simulink model "clearing_faulted_segment_travelling_Wave"  (R2018a)
settings: Solver=ode23t  StartTime=0.0  StopTime=2  MaxStep=1e-3  RelTol=1e-3
values from neighbouring files (symbols this model uses):
  AC_lim = [1.5 -1.5]    [MT_HVDC_initialize.m]
  C_pm = 10.48e-3    (= 0.01048)    [MT_HVDC_initialize.m]
  ccsc_lim = [1.0 -1.0]    [MT_HVDC_initialize.m]
  DC_lim = [1.05 -1.05]    [MT_HVDC_initialize.m]
  f = 50    [MT_HVDC_initialize.m]
  Fc = 50    [MT_HVDC_initialize.m]
  Fn_filter = 1000    [MT_HVDC_initialize.m]
  Ireg_lim_i = [1.5, -1.5]    [MT_HVDC_initialize.m]
  Ireg_lim_r = [1.5, -1.5]    [MT_HVDC_initialize.m]
  Ki_ACreg_i = 260    [MT_HVDC_initialize.m]
  Ki_ccsc = 5    [MT_HVDC_initialize.m]
  Ki_DCreg_r = 150    [MT_HVDC_initialize.m]
  Ki_Ireg_i = 200    [MT_HVDC_initialize.m]
  Ki_Ireg_r = 100    [MT_HVDC_initialize.m]
  Ki_R_inv = 150000    [MT_HVDC_initialize.m]
  Ki_R_rec = 5000    [MT_HVDC_initialize.m]
  Kp_ACreg_i = 2    [MT_HVDC_initialize.m]
  Kp_ccsc = 1    [MT_HVDC_initialize.m]
  Kp_DCreg_r = 8    [MT_HVDC_initialize.m]
  Kp_Ireg_i = 2    [MT_HVDC_initialize.m]
  Kp_Ireg_r = 2    [MT_HVDC_initialize.m]
  Kp_R_inv = 0.001    [MT_HVDC_initialize.m]
  Kp_R_rec = 0.001    [MT_HVDC_initialize.m]
  L1_pu = 0.109    [MT_HVDC_initialize.m]
  L2_pu = 0.0824    [MT_HVDC_initialize.m]
  L_arm = L_arm_pu*Z_base66/w    [MT_HVDC_initialize.m]
  L_arm_pu = 0.15    [MT_HVDC_initialize.m]
  L_int = X_int/w    [MT_HVDC_initialize.m]
  n = 50    [MT_HVDC_initialize.m]
  n2 = 50    [MT_HVDC_initialize.m]
  P_nom = 220e6    (= 220000000)    [MT_HVDC_initialize.m]
  R1_pu = 0.00206    [MT_HVDC_initialize.m]
  R2_pu = 0.00206    [MT_HVDC_initialize.m]
  R_arm = 0.03    [MT_HVDC_initialize.m]
  R_arm_pu = R_arm/Z_base66    [MT_HVDC_initialize.m]
  R_int = sqrt((z_int_400^2)/(1+xr_ratio^2))    [MT_HVDC_initialize.m]
  Rg_T1 = 40    [MT_HVDC_initialize.m]
  S1_nom = P_nom    (= 220000000)    [MT_HVDC_initialize.m]
  S2_nom = P_nom    (= 220000000)    [MT_HVDC_initialize.m]
  T_fault = 1.4    [MT_HVDC_initialize.m]
  Ts_Control = 40e-6    (= 4e-05)    [MT_HVDC_initialize.m]
  Ts_Power = 20e-6    (= 2e-05)    [MT_HVDC_initialize.m]
  V1_prim = V_prim    (= 400000)    [MT_HVDC_initialize.m]
  V1_sec = V_grid    (= 66000)    [MT_HVDC_initialize.m]
  V2_prim = V_grid    (= 66000)    [MT_HVDC_initialize.m]
  V2_sec = 18e3    (= 18000)    [MT_HVDC_initialize.m]
  V_ac_ref = 1.035    [MT_HVDC_initialize.m]
  V_grid = 66e3    (= 66000)    [MT_HVDC_initialize.m]
  V_prim = 400e3    (= 400000)    [MT_HVDC_initialize.m]
  Vc_pm_r = 0*Vdc_nom/n    (= 0)    [MT_HVDC_initialize.m]
  Vdc_nom = 135e3    (= 135000)    [MT_HVDC_initialize.m]
  w = 2*pi*f    (= 314.159265359)    [MT_HVDC_initialize.m]
  z0z1 = 0.8    [MT_HVDC_initialize.m]
  Zeta_filter = 1    [MT_HVDC_initialize.m]
undefined symbols (not defined in the file or in its folder): D1, Delta, DiscIntNeverNeededParam
libraries: powerlib x417, powerlib_meascontrol x130, simulink x84, powerlib_extras x8, simulink_extras x5
(part 13 of 17)

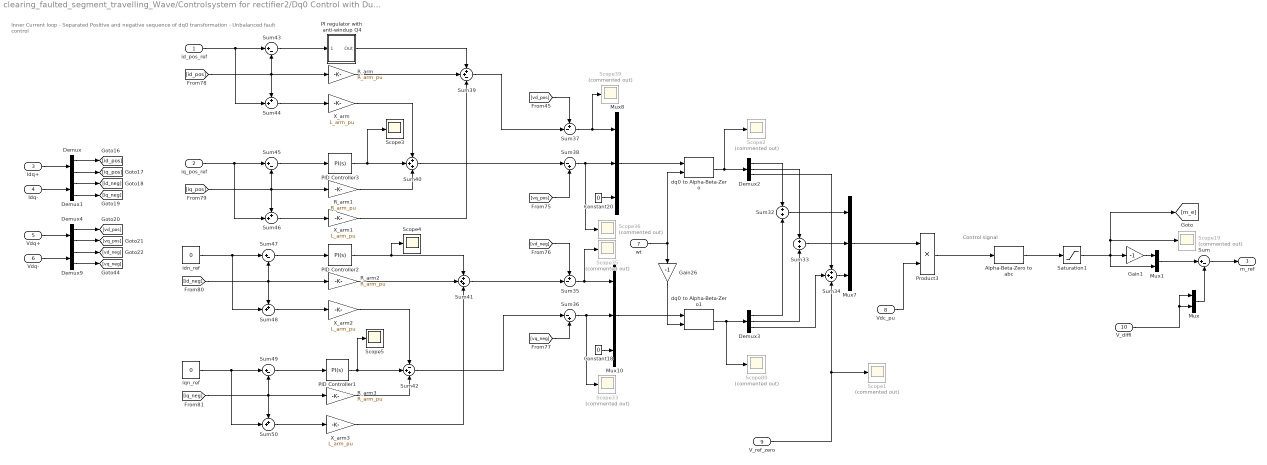
== system clearing_faulted_segment_travelling_Wave/Controlsystem for rectifier2/Dq0 Control with Dual Synchronous Reference Frame (DSRF)/Inner Current loop - Positive and Negative Sequence Control - Rectifier ==
  note: Control signal
  note: Inner Current loop - Separated Positive and negative sequence of dq0 transformation - Unbalanced fault control
  id_pos_ref : Inport
  iq_pos_ref : Inport  Port=2
  Idq+ : Inport  Port=3
  Idq- : Inport  Port=4
  Vdq+ : Inport  Port=5
  Vdq- : Inport  Port=6
  wt : Inport  Port=7
  Vdc_pu : Inport  Port=8
  V_ref_zero : Inport  Port=9
  V_diffi : Inport  Port=10
  Alpha-Beta-Zero to abc : powerlib_meascontrol/Transformations/Alpha-Beta-Zero to abc
      settings: SourceProductName=Simscape Electrical  SourceProductBaseCode=PS
  Constant18 : Constant  Value=0
  Constant20 : Constant  Value=0
  Demux{,1,4,9} (4 alike) : Demux  Outputs=2
  Demux2 : Demux  Outputs=3
  Demux3 : Demux  Outputs=3
  Gain1 : Gain  Gain=-1
  Gain26 : Gain  Gain=-1
  Mux : Mux  Inputs=2
  Mux1 : Mux  Inputs=2
  Mux10 : Mux  Inputs=3
  Mux7 : Mux  Inputs=3
  Mux8 : Mux  Inputs=3
  PI regulator with anti-windup Q4 : Subsystem  DialogController=POWERSYS.PowerSysDialog  mask(Discrete PI Controller){Kp=Kp_Ireg_r, Ki=Ki_Ireg_r, Par_Limits=[Ireg_lim_r(1) Ireg_lim_r(2)], Init=0, Ts=Ts_Control}
      mask prompts: Kp "Proportional gain (Kp):"; Ki "Integral gain (Ki):"; Par_Limits "Output limits: [ Upper   Lower ]"; Init "Output initial value:"; Ts "Sample time:"
      mask help: This block implements a discrete PI controller.
      mask init:
      | UpperLimit=Par_Limits(1);
      | LowerLimit=Par_Limits(2);
      | power_initmask();
      mask Help: This block is part of a subset of blocks in the Extras library that does not have documentation associated with it, other than the block mask description.
      mask Display: disp('PI');
  PID Controller1 : simulink/Continuous/PID Controller  Controller=PI  TimeDomain=Continuous-time  SampleTime=-1  IntegratorMethod=Forward Euler  FilterMethod=Forward Euler  Form=Parallel  UseFilter=on  ControllerParametersSource=internal  P=Kp_Ireg_r*0.5  I=Ki_Ireg_r*0.5  D=0  N=100  InitialConditionSource=internal  InitialConditionForIntegrator=0  InitialConditionForFilter=0  ExternalReset=none  LimitOutput=off  UpperSaturationLimit=inf  LowerSaturationLimit=-inf  LinearizeAsGain=on  AntiWindupMode=none  Kb=1  TrackingMode=off  Kt=1  PParamMin=[]  PParamMax=[]  IParamMin=[]  IParamMax=[]  DParamMin=[]  DParamMax=[]  NParamMin=[]  NParamMax=[]  KbParamMin=[]  KbParamMax=[]  KtParamMin=[]  KtParamMax=[]  POutMin=[]  POutMax=[]  IOutMin=[]  IOutMax=[]  DOutMin=[]  DOutMax=[]  NOutMin=[]  NOutMax=[]  KbOutMin=[]  KbOutMax=[]  KtOutMin=[]  KtOutMax=[]  IntegratorOutMin=[]  IntegratorOutMax=[]  FilterOutMin=[]  FilterOutMax=[]  SumOutMin=[]  SumOutMax=[]  SumI1OutMin=[]  SumI1OutMax=[]  SumI2OutMin=[]  SumI2OutMax=[]  SumI3OutMin=[]  SumI3OutMax=[]  SumDOutMin=[]  SumDOutMax=[]  SaturationOutMin=[]  SaturationOutMax=[]  IntegratorContinuousStateAttributes=''  IntegratorStateMustResolveToSignalObject=off  IntegratorRTWStateStorageClass=Auto  FilterContinuousStateAttributes=''  FilterStateMustResolveToSignalObject=off  FilterRTWStateStorageClass=Auto  DifferentiatorICPrevScaledInput=0  DifferentiatorOutMin=[]  DifferentiatorOutMax=[]  FilterDiffOutCoefMin=[]  FilterDiffOutCoefMax=[]  SumDenOutMin=[]  SumDenOutMax=[]  SumNumOutMin=[]  SumNumOutMax=[]  ReciprocalOutMin=[]  ReciprocalOutMax=[]  DivideOutMin=[]  DivideOutMax=[]  TunerSelectOption=Transfer Function Based (PID Tuner App)
  PID Controller2 : simulink/Continuous/PID Controller  Controller=PI  TimeDomain=Continuous-time  SampleTime=-1  IntegratorMethod=Forward Euler  FilterMethod=Forward Euler  Form=Parallel  UseFilter=on  ControllerParametersSource=internal  P=Kp_Ireg_r*0.5  I=Ki_Ireg_r*0.5  D=0  N=100  InitialConditionSource=internal  InitialConditionForIntegrator=0  InitialConditionForFilter=0  ExternalReset=none  LimitOutput=off  UpperSaturationLimit=inf  LowerSaturationLimit=-inf  LinearizeAsGain=on  AntiWindupMode=none  Kb=1  TrackingMode=off  Kt=1  PParamMin=[]  PParamMax=[]  IParamMin=[]  IParamMax=[]  DParamMin=[]  DParamMax=[]  NParamMin=[]  NParamMax=[]  KbParamMin=[]  KbParamMax=[]  KtParamMin=[]  KtParamMax=[]  POutMin=[]  POutMax=[]  IOutMin=[]  IOutMax=[]  DOutMin=[]  DOutMax=[]  NOutMin=[]  NOutMax=[]  KbOutMin=[]  KbOutMax=[]  KtOutMin=[]  KtOutMax=[]  IntegratorOutMin=[]  IntegratorOutMax=[]  FilterOutMin=[]  FilterOutMax=[]  SumOutMin=[]  SumOutMax=[]  SumI1OutMin=[]  SumI1OutMax=[]  SumI2OutMin=[]  SumI2OutMax=[]  SumI3OutMin=[]  SumI3OutMax=[]  SumDOutMin=[]  SumDOutMax=[]  SaturationOutMin=[]  SaturationOutMax=[]  IntegratorContinuousStateAttributes=''  IntegratorStateMustResolveToSignalObject=off  IntegratorRTWStateStorageClass=Auto  FilterContinuousStateAttributes=''  FilterStateMustResolveToSignalObject=off  FilterRTWStateStorageClass=Auto  DifferentiatorICPrevScaledInput=0  DifferentiatorOutMin=[]  DifferentiatorOutMax=[]  FilterDiffOutCoefMin=[]  FilterDiffOutCoefMax=[]  SumDenOutMin=[]  SumDenOutMax=[]  SumNumOutMin=[]  SumNumOutMax=[]  ReciprocalOutMin=[]  ReciprocalOutMax=[]  DivideOutMin=[]  DivideOutMax=[]  TunerSelectOption=Transfer Function Based (PID Tuner App)
  PID Controller3 : simulink/Continuous/PID Controller  Controller=PI  TimeDomain=Continuous-time  SampleTime=-1  IntegratorMethod=Forward Euler  FilterMethod=Forward Euler  Form=Parallel  UseFilter=on  ControllerParametersSource=internal  P=Kp_Ireg_r  I=Ki_Ireg_r  D=0  N=100  InitialConditionSource=internal  InitialConditionForIntegrator=0  InitialConditionForFilter=0  ExternalReset=none  LimitOutput=off  UpperSaturationLimit=inf  LowerSaturationLimit=-inf  LinearizeAsGain=on  AntiWindupMode=none  Kb=1  TrackingMode=off  Kt=1  PParamMin=[]  PParamMax=[]  IParamMin=[]  IParamMax=[]  DParamMin=[]  DParamMax=[]  NParamMin=[]  NParamMax=[]  KbParamMin=[]  KbParamMax=[]  KtParamMin=[]  KtParamMax=[]  POutMin=[]  POutMax=[]  IOutMin=[]  IOutMax=[]  DOutMin=[]  DOutMax=[]  NOutMin=[]  NOutMax=[]  KbOutMin=[]  KbOutMax=[]  KtOutMin=[]  KtOutMax=[]  IntegratorOutMin=[]  IntegratorOutMax=[]  FilterOutMin=[]  FilterOutMax=[]  SumOutMin=[]  SumOutMax=[]  SumI1OutMin=[]  SumI1OutMax=[]  SumI2OutMin=[]  SumI2OutMax=[]  SumI3OutMin=[]  SumI3OutMax=[]  SumDOutMin=[]  SumDOutMax=[]  SaturationOutMin=[]  SaturationOutMax=[]  IntegratorContinuousStateAttributes=''  IntegratorStateMustResolveToSignalObject=off  IntegratorRTWStateStorageClass=Auto  FilterContinuousStateAttributes=''  FilterStateMustResolveToSignalObject=off  FilterRTWStateStorageClass=Auto  DifferentiatorICPrevScaledInput=0  DifferentiatorOutMin=[]  DifferentiatorOutMax=[]  FilterDiffOutCoefMin=[]  FilterDiffOutCoefMax=[]  SumDenOutMin=[]  SumDenOutMax=[]  SumNumOutMin=[]  SumNumOutMax=[]  ReciprocalOutMin=[]  ReciprocalOutMax=[]  DivideOutMin=[]  DivideOutMax=[]  TunerSelectOption=Transfer Function Based (PID Tuner App)
  Product3 : Product
  R_arm{,1..3} (4 alike) : Gain  Gain=R_arm_pu
  Saturation1 : Saturate  UpperLimit=Ireg_lim_r(1) + 1.1*0  LowerLimit=Ireg_lim_r(2)
  Scope{1..2,19,33,35..36,39,80} (8 alike) : Scope  Commented=on
  Scope3 : Scope
  Scope4 : Scope
  Scope5 : Scope
  Sum{,43,45,47,49} (5 alike) : Sum  Inputs=|+-
  Sum32 : Sum
  Sum33 : Sum
  Sum34 : Sum  Inputs=+++
  Sum35 : Sum  Inputs=+-|
  Sum36 : Sum  Inputs=|-+
  Sum37 : Sum  Inputs=+-|
  Sum38 : Sum  Inputs=|-+
  Sum39 : Sum  Inputs=++-
  Sum40 : Sum  Inputs=+++
  Sum41 : Sum  Inputs=+++
  Sum42 : Sum  Inputs=-++
  Sum{44,46,48,50} (4 alike) : Sum  Inputs=++|
  X_arm{,1..3} (4 alike) : Gain  Gain=L_arm_pu
  dq0 to Alpha-Beta-Zero : powerlib_meascontrol/Transformations/dq0 to Alpha-Beta-Zero  Alignment=90 degrees behind phase A axis
      settings: SourceProductName=Simscape Electrical  SourceProductBaseCode=PS
  dq0 to Alpha-Beta-Zero1 : powerlib_meascontrol/Transformations/dq0 to Alpha-Beta-Zero  Alignment=90 degrees behind phase A axis
      settings: SourceProductName=Simscape Electrical  SourceProductBaseCode=PS
  idn_ref : Constant  Value=0
  iqn_ref : Constant  Value=0
  m_ref : Outport
  wires:
  Vdq-/1 -> Demux9/1
  Idq-/1 -> Demux1/1
  Vdq+/1 -> Demux4/1
  Demux9/2 -> [vq_neg]
  Demux1/1 -> [id_neg]
  Demux4/2 -> [vq_pos]
  Demux4/1 -> [vd_pos]
  Demux/1 -> [id_pos]
  Demux/2 -> [iq_pos]
  wt/1 -> Gain26/1, dq0 to Alpha-Beta-Zero/2
  Sum36/1 -> Mux10/2, Scope33/1
  Sum45/1 -> PID Controller3/1
  Sum37/1 -> Mux8/1, Scope39/1
  V_ref_zero/1 -> Scope1/1, Sum34/3
  X_arm3/1 -> Sum41/3
  X_arm2/1 -> Sum42/1
  iq_pos_ref/1 -> Sum45/1, Sum46/2
  idn_ref/1 -> Sum47/1, Sum48/2
  Demux3/1 -> Sum32/2
  Sum40/1 -> Sum38/1
  X_arm1/1 -> Sum39/3
  [vq_neg] -> Sum36/2
  R_arm1/1 -> Sum40/3
  Sum48/1 -> X_arm2/1
  R_arm/1 -> Sum39/2
  Sum44/1 -> X_arm/1
  Sum43/1 -> PI regulator with anti-windup Q4/1(Error)
  Sum46/1 -> X_arm1/1
  Product3/1 -> Alpha-Beta-Zero to abc/1
  Sum38/1 -> Scope36/1, Mux8/2
  [vd_pos] -> Sum37/1
  iqn_ref/1 -> Sum49/1, Sum50/2
  Idq+/1 -> Demux/1
  [vd_neg] -> Sum35/1
  Sum47/1 -> PID Controller2/1
  [vq_pos] -> Sum38/2
  X_arm/1 -> Sum40/1
  Sum33/1 -> Mux7/2
  R_arm3/1 -> Sum42/3
  Sum41/1 -> Sum35/2
  Demux2/1 -> Sum32/1
  Sum42/1 -> Sum36/1
  Sum39/1 -> Sum37/2
  id_pos_ref/1 -> Sum43/1, Sum44/2
  [iq_neg] -> Sum49/2, Sum50/1, R_arm3/1
  Demux3/3 -> Sum34/2
  [id_neg] -> Sum48/1, Sum47/2, R_arm2/1
  Sum35/1 -> Mux10/1, Scope35/1
  [id_pos] -> Sum44/1, Sum43/2, R_arm/1
  Constant20/1 -> Mux8/3
  Constant18/1 -> Mux10/3
  Demux2/2 -> Sum33/1
  Demux2/3 -> Sum34/1
  Sum50/1 -> X_arm3/1
  Sum49/1 -> PID Controller1/1
  [iq_pos] -> Sum45/2, Sum46/1, R_arm1/1
  Sum34/1 -> Mux7/3
  Demux3/2 -> Sum33/2
  R_arm2/1 -> Sum41/2
  dq0 to Alpha-Beta-Zero/1 -> Demux2/1, Scope2/1
  Sum32/1 -> Mux7/1
  Gain26/1 -> dq0 to Alpha-Beta-Zero1/2
  Demux1/2 -> [iq_neg]
  dq0 to Alpha-Beta-Zero1/1 -> Demux3/1, Scope80/1
  Demux9/1 -> [vd_neg]
  Alpha-Beta-Zero to abc/1 -> Saturation1/1
  Mux10/1 -> dq0 to Alpha-Beta-Zero1/1
  Mux8/1 -> dq0 to Alpha-Beta-Zero/1
  Mux7/1 -> Product3/1
  Vdc_pu/1 -> Product3/2
  PID Controller3/1 -> Sum40/2, Scope3/1
  PID Controller2/1 -> Sum41/1, Scope4/1
  PID Controller1/1 -> Sum42/2, Scope5/1
  PI regulator with anti-windup Q4/1(Out) -> Sum39/1
  V_diffi/1 -> Mux/1, Mux/2
  Mux/1 -> Sum/2
  Mux1/1 -> Sum/1
  Sum/1 -> m_ref/1
  Saturation1/1 -> Gain1/1, Mux1/2, Scope19/1, [m_e]
  Gain1/1 -> Mux1/1

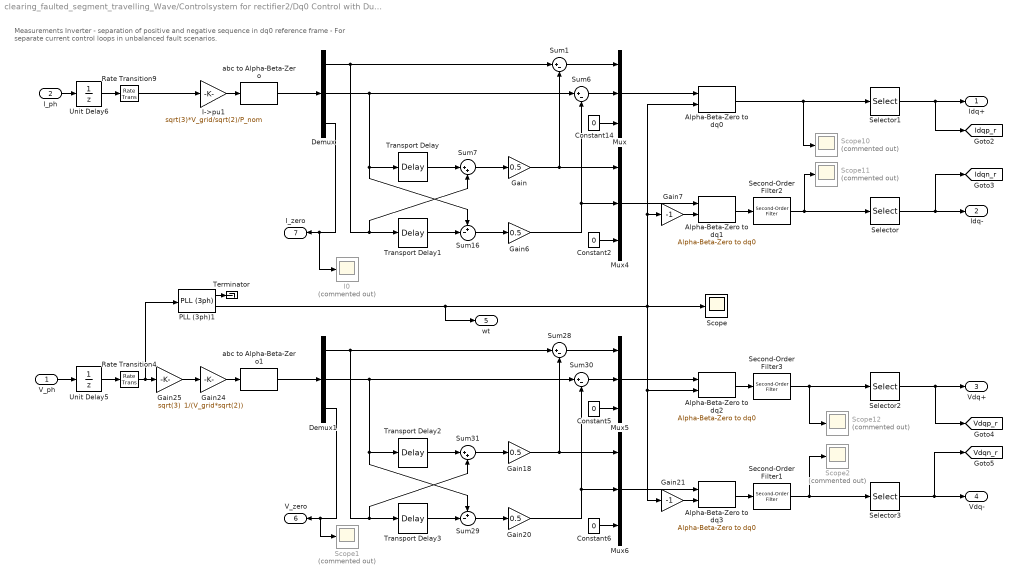
== system clearing_faulted_segment_travelling_Wave/Controlsystem for rectifier2/Dq0 Control with Dual Synchronous Reference Frame (DSRF)/Measurement - dq0 positiveand negative sequence, - and zero sequence in alphabetta - Rectifier ==
  note: Measurements Inverter - separation of positive and negative sequence in dq0 reference frame - For separate current control loops in unbalanced fault scenarios.
  V_ph : Inport
  I_ph : Inport  Port=2
  Alpha-Beta-Zero to dq{0..3} (4 alike) : powerlib_meascontrol/Transformations/Alpha-Beta-Zero to dq0  Alignment=90 degrees behind phase A axis
      settings: SourceProductName=Simscape Electrical
  Constant{2,5..6,14} (4 alike) : Constant  Value=0
  Demux : Demux  Outputs=3
  Demux1 : Demux  Outputs=3
  Gain{,6,18,20} (4 alike) : Gain  Gain=0.5
  Gain21 : Gain  Gain=-1
  Gain24 : Gain  Gain=1/(V_grid*sqrt(2))
  Gain25 : Gain  Gain=sqrt(3)
  Gain7 : Gain  Gain=-1
  I->pu1 : Gain  Gain=sqrt(3)*V_grid/sqrt(2)/P_nom  SaturateOnIntegerOverflow=on  OutDataTypeStr=Inherit: Same as input  ParamDataTypeStr=Inherit: Same as input
  "I0 " : Scope  Commented=on
  Mux{,4..6} (4 alike) : Mux  Inputs=3
  PLL (3ph)1 : powerlib_meascontrol/PLL/PLL (3ph)  Fmin=45  Par_Init=[V_grid, f]  ParK=[180, 3200, 1]  TcD=1e-4  MaxRateChangeFreq=12  FilterCutOffFreq=25  Ts=0  AGC=on
      settings: SourceProductName=Simscape Electrical
  Rate Transition4 : RateTransition  OutPortSampleTime=Ts_Control
  Rate Transition9 : RateTransition  OutPortSampleTime=Ts_Control
  Scope : Scope
  Scope{1..2,10..12} (5 alike) : Scope  Commented=on
  Second-Order Filter1 : powerlib_meascontrol/Filters/Second-Order Filter  FilterType=Bandstop (Notch)  Fo=100  Zeta=Zeta_filter*0.8  Ts=Ts_Control  Initialize=off  Vac_Init="[0,  0,  60]"  Vdc_Init=0  PlotResponse=off  FreqRange=[0, 500, 1]
      settings: SourceProductName=Simscape Electrical  SourceProductBaseCode=PS
  Second-Order Filter2 : powerlib_meascontrol/Filters/Second-Order Filter  FilterType=Bandstop (Notch)  Fo=100  Zeta=Zeta_filter*0.8  Ts=Ts_Control  Initialize=off  Vac_Init="[0,  0,  60]"  Vdc_Init=0  PlotResponse=off  FreqRange=[0, 500, 1]
      settings: SourceProductName=Simscape Electrical  SourceProductBaseCode=PS
  Second-Order Filter3 : powerlib_meascontrol/Filters/Second-Order Filter  FilterType=Lowpass  Fo=Fn_filter  Zeta=Zeta_filter  Ts=Ts_Control  Initialize=off  Vac_Init="[0,  0,  60]"  Vdc_Init=0  PlotResponse=off  FreqRange=[0, 500, 1]
      settings: SourceProductName=Simscape Electrical  SourceProductBaseCode=PS
  Selector{,1..3} (4 alike) : Selector  InputPortWidth=3  IndexOptions=Index vector (dialog)  Indices=[1 2]  OutputSizes=1
  Sum{1,6,28,30} (4 alike) : Sum  Inputs=|+-
  Sum16 : Sum  Inputs=+-|
  Sum29 : Sum  Inputs=+-|
  Sum31 : Sum  Inputs=|++
  Sum7 : Sum  Inputs=|++
  Terminator : Terminator
  Transport Delay{,1..3} (4 alike) : TransportDelay  DelayTime=1/(f*4)  BufferSize=1024*15
  Unit Delay5 : UnitDelay  SampleTime=Ts_Power
  Unit Delay6 : UnitDelay  SampleTime=Ts_Power
  abc to Alpha-Beta-Zero : powerlib_meascontrol/Transformations/abc to Alpha-Beta-Zero
      settings: SourceProductName=Simscape Electrical
  abc to Alpha-Beta-Zero1 : powerlib_meascontrol/Transformations/abc to Alpha-Beta-Zero
      settings: SourceProductName=Simscape Electrical
  Idq+ : Outport
  Idq- : Outport  Port=2
  Vdq+ : Outport  Port=3
  Vdq- : Outport  Port=4
  wt : Outport  Port=5
  V_zero : Outport  Port=6
  I_zero : Outport  Port=7
  tag scope: Idqn_r=global, Idqp_r=global, Vdqn_r=global, Vdqp_r=global
  wires:
  Selector2/1 -> [Vdqp_r], Vdq+/1
  Selector1/1 -> [Idqp_r], Idq+/1
  Sum29/1 -> Gain20/1
  Constant6/1 -> Mux6/3
  Sum1/1 -> Mux/1
  Sum7/1 -> Gain/1
  Gain7/1 -> Alpha-Beta-Zero to dq1/2
  Gain21/1 -> Alpha-Beta-Zero to dq3/2
  I_ph/1 -> Unit Delay6/1
  Sum30/1 -> Mux5/2
  Demux/3 -> "I0 "/1, I_zero/1
  Mux4/1 -> Alpha-Beta-Zero to dq1/1
  Rate Transition9/1 -> I->pu1/1
  Transport Delay3/1 -> Sum29/2
  Demux/2 -> Sum6/1, Transport Delay/1, Sum16/1
  Constant2/1 -> Mux4/3
  Gain25/1 -> Gain24/1
  Gain24/1 -> abc to Alpha-Beta-Zero1/1
  I->pu1/1 -> abc to Alpha-Beta-Zero/1
  Unit Delay6/1 -> Rate Transition9/1
  Sum31/1 -> Gain18/1
  Unit Delay5/1 -> Rate Transition4/1
  Mux5/1 -> Alpha-Beta-Zero to dq2/1
  Sum28/1 -> Mux5/1
  Transport Delay2/1 -> Sum31/1
  Gain20/1 -> Sum30/2, Mux6/2
  Constant5/1 -> Mux5/3
  Mux6/1 -> Alpha-Beta-Zero to dq3/1
  Transport Delay/1 -> Sum7/1
  Sum6/1 -> Mux/2
  Gain18/1 -> Sum28/2, Mux6/1
  Gain/1 -> Mux4/1, Sum1/2
  Gain6/1 -> Mux4/2, Sum6/2
  Demux/1 -> Sum1/1, Sum7/2, Transport Delay1/1
  Demux1/3 -> Scope1/1, V_zero/1
  Transport Delay1/1 -> Sum16/2
  Mux/1 -> Alpha-Beta-Zero to dq0/1
  abc to Alpha-Beta-Zero/1 -> Demux/1
  Demux1/1 -> Transport Delay3/1, Sum31/2, Sum28/1
  abc to Alpha-Beta-Zero1/1 -> Demux1/1
  Demux1/2 -> Sum29/1, Transport Delay2/1, Sum30/1
  Sum16/1 -> Gain6/1
  Constant14/1 -> Mux/3
  Rate Transition4/1 -> PLL (3ph)1/1, Gain25/1
  PLL (3ph)1/2 -> wt/1, Gain7/1, Alpha-Beta-Zero to dq0/2, Scope/1, Alpha-Beta-Zero to dq2/2, Gain21/1
  V_ph/1 -> Unit Delay5/1
  PLL (3ph)1/1 -> Terminator/1
  Alpha-Beta-Zero to dq3/1 -> Second-Order Filter1/1
  Alpha-Beta-Zero to dq1/1 -> Second-Order Filter2/1
  Selector3/1 -> [Vdqn_r], Vdq-/1
  Selector/1 -> [Idqn_r], Idq-/1
  Alpha-Beta-Zero to dq0/1 -> Scope10/1, Selector1/1
  Alpha-Beta-Zero to dq2/1 -> Second-Order Filter3/1
  Second-Order Filter1/1 -> Scope2/1, Selector3/1
  Second-Order Filter3/1 -> Selector2/1, Scope12/1
  Second-Order Filter2/1 -> Scope11/1, Selector/1

== system clearing_faulted_segment_travelling_Wave/Controlsystem for rectifier2/Dq0 Control with Dual Synchronous Reference Frame (DSRF)/PWM Signal Generator - Rectifier ==
  U_ref : Inport
  Block : Inport  Port=2
  Add{,7..11} (6 alike) : Sum  Inputs=1
  Constant{3..8} (6 alike) : Constant  Value=0
  Constant9 : Constant  Value=[ 0, n ]
  Demux : Demux  Outputs=2
  Demux1 : Demux  Outputs=3
  Demux4 : Demux  Outputs=3
  Mux{7..12} (6 alike) : Mux  Inputs=2
  Mux13 : Mux  Inputs=6
  PWM Gen1 : Subsystem  mask(PWM generator for half-bridge MMC){n=n, Fc=Fc, Ts=Ts_Power}
      mask prompts: n "Number of half-bridges"; Fc "Carriers frequency (Hz)"; Ts "Sample time (s)"
      mask init: same as clearing_faulted_segment_travelling_Wave/Controlsystem for Inverter/Dq0 Control/PWM Signal Generator - Inverter1/PWM Gen1
  PWM Gen2 : Subsystem  mask(PWM generator for half-bridge MMC){n=n, Fc=Fc, Ts=Ts_Power}
      mask prompts: n "Number of half-bridges"; Fc "Carriers frequency (Hz)"; Ts "Sample time (s)"
      mask init: same as clearing_faulted_segment_travelling_Wave/Controlsystem for Inverter/Dq0 Control/PWM Signal Generator - Inverter1/PWM Gen1
  PWM Gen3 : Subsystem  mask(PWM generator for half-bridge MMC){n=n, Fc=Fc, Ts=Ts_Power}
      mask prompts: n "Number of half-bridges"; Fc "Carriers frequency (Hz)"; Ts "Sample time (s)"
      mask init: same as clearing_faulted_segment_travelling_Wave/Controlsystem for Inverter/Dq0 Control/PWM Signal Generator - Inverter1/PWM Gen1
  PWM Gen4 : Subsystem  mask(PWM generator for half-bridge MMC){n=n, Fc=Fc, Ts=Ts_Power}
      mask prompts: n "Number of half-bridges"; Fc "Carriers frequency (Hz)"; Ts "Sample time (s)"
      mask init: same as clearing_faulted_segment_travelling_Wave/Controlsystem for Inverter/Dq0 Control/PWM Signal Generator - Inverter1/PWM Gen1
  PWM Gen5 : Subsystem  mask(PWM generator for half-bridge MMC){n=n, Fc=Fc, Ts=Ts_Power}
      mask prompts: n "Number of half-bridges"; Fc "Carriers frequency (Hz)"; Ts "Sample time (s)"
      mask init: same as clearing_faulted_segment_travelling_Wave/Controlsystem for Inverter/Dq0 Control/PWM Signal Generator - Inverter1/PWM Gen1
  PWM Gen6 : Subsystem  mask(PWM generator for half-bridge MMC){n=n, Fc=Fc, Ts=Ts_Power}
      mask prompts: n "Number of half-bridges"; Fc "Carriers frequency (Hz)"; Ts "Sample time (s)"
      mask init: same as clearing_faulted_segment_travelling_Wave/Controlsystem for Inverter/Dq0 Control/PWM Signal Generator - Inverter1/PWM Gen1
  Selector{,1..5} (6 alike) : Selector  InputPortWidth=n*2  IndexOptions=Index vector (dialog)  Indices=[1:2:(n*2-1)]  OutputSizes=1
  Switch{,1..5} (6 alike) : Switch  Criteria=u2 ~= 0
  Terminator{,1..5} (6 alike) : Terminator
  g : Outport
  wires:
  Selector5/1 -> Add11/1
  Switch3/1 -> Mux13/4
  Switch4/1 -> Mux13/5
  PWM Gen1/1(P) -> Selector/1
  Demux4/3 -> PWM Gen3/1(Uref)
  Switch2/1 -> Mux13/3
  PWM Gen4/2(Cr) -> Terminator4/1
  Switch/1 -> Mux13/1
  Mux13/1 -> g/1
  Constant4/1 -> Mux8/2
  Demux1/3 -> PWM Gen6/1(Uref)
  Mux10/1 -> Switch3/3
  Mux8/1 -> Switch1/3
  Selector3/1 -> Add9/1
  Constant8/1 -> Mux12/2
  Selector4/1 -> Add10/1
  Constant6/1 -> Mux10/2
  Constant5/1 -> Mux9/2
  Selector1/1 -> Add7/1
  Demux1/1 -> PWM Gen4/1(Uref)
  Add9/1 -> Mux10/1
  Demux4/1 -> PWM Gen1/1(Uref)
  Selector2/1 -> Add8/1
  Add7/1 -> Mux8/1
  Constant9/1 -> Switch/1, Switch5/1, Switch4/1, Switch3/1, Switch2/1, Switch1/1
  PWM Gen3/2(Cr) -> Terminator1/1
  PWM Gen5/1(P) -> Selector4/1
  Constant7/1 -> Mux11/2
  Demux4/2 -> PWM Gen2/1(Uref)
  Mux12/1 -> Switch5/3
  PWM Gen6/2(Cr) -> Terminator3/1
  PWM Gen2/2(Cr) -> Terminator/1
  Switch5/1 -> Mux13/6
  Selector/1 -> Add/1
  Block/1 -> Switch/2, Switch1/2, Switch2/2, Switch3/2, Switch4/2, Switch5/2
  Add10/1 -> Mux11/1
  PWM Gen5/2(Cr) -> Terminator2/1
  Add11/1 -> Mux12/1
  Demux1/2 -> PWM Gen5/1(Uref)
  Mux11/1 -> Switch4/3
  Mux7/1 -> Switch/3
  Switch1/1 -> Mux13/2
  Constant3/1 -> Mux7/2
  PWM Gen4/1(P) -> Selector3/1
  PWM Gen2/1(P) -> Selector1/1
  Mux9/1 -> Switch2/3
  PWM Gen3/1(P) -> Selector2/1
  Add8/1 -> Mux9/1
  Add/1 -> Mux7/1
  PWM Gen6/1(P) -> Selector5/1
  PWM Gen1/2(Cr) -> Terminator5/1
  U_ref/1 -> Demux/1
  Demux/1 -> Demux4/1
  Demux/2 -> Demux1/1

== system clearing_faulted_segment_travelling_Wave/Controlsystem for rectifier2/Dq0 Control with Dual Synchronous Reference Frame (DSRF)/Zero Sequence Controller2 ==
  note: PR Controller
  V0_meas : Inport
  I0_meas : Inport  Port=2
  Enable : Inport  Port=3
  Enable1 : EnablePort
  Constant : Constant  Value=0
  Constant1 : Constant  Value=0
  I0_r_ref : Constant  Value=0
  Ki_R : Gain  Gain=Ki_R_rec
  Kp_R : Gain  Gain=Kp_R_rec
  Second-Order Filter1 : powerlib_meascontrol/Filters/Second-Order Filter  FilterType=Lowpass  Fo=f*4  Zeta=0.707  Ts=0  Initialize=on  Vac_Init="[0,  0,  60]"  Vdc_Init=0  PlotResponse=off  FreqRange=[0, 500, 1]
      settings: SourceProductName=Simscape Electrical  SourceProductBaseCode=PS
  Second-Order Filter2 : powerlib_meascontrol/Filters/Second-Order Filter  FilterType=Bandstop (Notch)  Fo=f*2  Zeta=0.707  Ts=0  Initialize=off  Vac_Init="[0,  0,  60]"  Vdc_Init=0  PlotResponse=off  FreqRange=[0, 500, 1]
      settings: SourceProductName=Simscape Electrical  SourceProductBaseCode=PS
  Sum2 : Sum  Inputs=+-|
  Sum3 : Sum  Inputs=++|
  Sum96 : Sum  Inputs=|++
  Switch : Switch  Criteria=u2 > Threshold
  Switch1 : Switch  Criteria=u2 > Threshold
  Transfer Fcn1 : TransferFcn  Denominator=[1 0 98596]
  V_zero_ref : Outport
  wires:
  I0_r_ref/1 -> Sum2/1
  Kp_R/1 -> Sum96/1
  Sum96/1 -> Sum3/2
  Switch/1 -> V_zero_ref/1
  Transfer Fcn1/1 -> Sum96/2
  Ki_R/1 -> Transfer Fcn1/1
  V0_meas/1 -> Second-Order Filter1/1
  Second-Order Filter1/1 -> Sum3/1
  Sum3/1 -> Switch/1
  Second-Order Filter2/1 -> Ki_R/1
  Sum2/1 -> Kp_R/1, Second-Order Filter2/1
  I0_meas/1 -> Switch1/1
  Switch1/1 -> Sum2/2
  Enable/1 -> Switch/2, Switch1/2
  Constant/1 -> Switch/3
  Constant1/1 -> Switch1/3

== system clearing_faulted_segment_travelling_Wave/MMC Converter1/Half-Bridge MMC Ap/HalfBridgeMMC_Agt_Discrete ==
  N : Inport  PortDimensions=2
  Current Measurement1 : powerlib/Measurements/Current Measurement  PhasorSimulation=off  OutputType=Complex  PSBequivalent=0
      settings: SourceProductName=Simscape Electrical
  Current Measurement2 : powerlib/Measurements/Current Measurement  PhasorSimulation=off  OutputType=Complex  PSBequivalent=0
      settings: SourceProductName=Simscape Electrical
  Demux : Demux  Outputs=2
  Discrete-Time Integrator : DiscreteIntegrator  IntegratorMethod=Integration: Trapezoidal  gainval=1  InitialCondition=Vc_Initial  SampleTime=Ts  UpperSaturationLimit=5000  LowerSaturationLimit=500  ICPrevOutput=DiscIntNeverNeededParam  ICPrevScaledInput=DiscIntNeverNeededParam
  Dp : powerlib/Power Electronics/Diode  Ron=Ron_Diode  Lon=0  Vf=Vf_Diode  IC=0  UseSnubber=off  Rs=Rs_Diode  Cs=Cs_Diode  Measurements=off
      settings: SourceProductName=Simscape Electrical
  Dp2 : powerlib/Power Electronics/Diode  Ron=Ron_Diode  Lon=0  Vf=Vf_Diode  IC=0  UseSnubber=off  Rs=Rs_Diode  Cs=Cs_Diode  Measurements=off
      settings: SourceProductName=Simscape Electrical
  Gain : Gain  Gain=1/(C*n)
  Gain2 : Gain  Gain=2
  Mux : Mux  Inputs=2
  Product1 : Product
  Product2 : Product
  Saturation1 : Saturate  UpperLimit=n  LowerLimit=0
  Sum1 : Sum  Inputs=1  SaturateOnIntegerOverflow=on  InputSameDT=on  OutDataTypeStr=Inherit: Same as first input
  Sum2 : Sum  Inputs=+-  SaturateOnIntegerOverflow=on  InputSameDT=on  OutDataTypeStr=Inherit: Same as first input
  Unit Delay1 : UnitDelay  SampleTime=Ts
  Unit Delay3 : UnitDelay  InitialCondition=Vc_Initial  SampleTime=Ts
  Unit Delay4 : UnitDelay  InitialCondition=Vc_Initial  SampleTime=Ts
  Vp : powerlib/Electrical Sources/Controlled Voltage Source  Initialize=off  Source_Type=AC  Amplitude=0  Phase=0  Frequency=0  Measurements=None
      settings: SourceProductName=Simscape Electrical
  Vp1 : powerlib/Electrical Sources/Controlled Voltage Source  Initialize=off  Source_Type=AC  Amplitude=0  Phase=0  Frequency=0  Measurements=None
      settings: SourceProductName=Simscape Electrical
  1 : PMIOPort  Side=Left
  2 : PMIOPort  Port=2  Side=Left
  Vc : Outport
  wires:
  N/1 -> Saturation1/1
  [Imod] -> Mux/1
  Unit Delay3/1 -> Sum2/2
  Unit Delay4/1 -> Unit Delay3/1, Gain2/1
  Gain2/1 -> Sum2/1
  Gain/1 -> Discrete-Time Integrator/1
  Discrete-Time Integrator/1 -> Unit Delay4/1
  Mux/1 -> Unit Delay1/1
  Product2/1 -> Demux/1
  Demux/1 -> [Vin]
  Demux/2 -> [Vbl]
  [Vin] -> Vp/1
  Current Measurement1/1 -> [Imod]
  Current Measurement2/1 -> [Icap]
  [Vbl] -> Vp1/1
  [Icap] -> Mux/2
  Unit Delay1/1 -> Product1/2
  Saturation1/1 -> Product1/1, Product2/1
  Product1/1 -> Sum1/1
  Sum2/1 -> Product2/2, Vc/1
  Sum1/1 -> Gain/1
  connections:
  1/RConn1 -- Vp/RConn1
  Vp/LConn1 -- Current Measurement1/LConn1
  Current Measurement1/RConn1 -- Dp/LConn1 -- Dp2/RConn1
  Current Measurement2/LConn1 -- Dp/RConn1
  Vp1/RConn1 -- Current Measurement2/RConn1
  Vp1/LConn1 -- 2/RConn1 -- Dp2/LConn1

== system clearing_faulted_segment_travelling_Wave/MMC Converter1/Half-Bridge MMC Ap1/HalfBridgeMMC_Agt_Discrete ==
  N : Inport  PortDimensions=2
  Current Measurement1 : powerlib/Measurements/Current Measurement  PhasorSimulation=off  OutputType=Complex  PSBequivalent=0
      settings: SourceProductName=Simscape Electrical
  Current Measurement2 : powerlib/Measurements/Current Measurement  PhasorSimulation=off  OutputType=Complex  PSBequivalent=0
      settings: SourceProductName=Simscape Electrical
  Demux : Demux  Outputs=2
  Discrete-Time Integrator : DiscreteIntegrator  IntegratorMethod=Integration: Trapezoidal  gainval=1  InitialCondition=Vc_Initial  SampleTime=Ts  UpperSaturationLimit=5000  LowerSaturationLimit=500  ICPrevOutput=DiscIntNeverNeededParam  ICPrevScaledInput=DiscIntNeverNeededParam
  Dp : powerlib/Power Electronics/Diode  Ron=Ron_Diode  Lon=0  Vf=Vf_Diode  IC=0  UseSnubber=off  Rs=Rs_Diode  Cs=Cs_Diode  Measurements=off
      settings: SourceProductName=Simscape Electrical
  Dp2 : powerlib/Power Electronics/Diode  Ron=Ron_Diode  Lon=0  Vf=Vf_Diode  IC=0  UseSnubber=off  Rs=Rs_Diode  Cs=Cs_Diode  Measurements=off
      settings: SourceProductName=Simscape Electrical
  Gain : Gain  Gain=1/(C*n)
  Gain2 : Gain  Gain=2
  Mux : Mux  Inputs=2
  Product1 : Product
  Product2 : Product
  Saturation1 : Saturate  UpperLimit=n  LowerLimit=0
  Sum1 : Sum  Inputs=1  SaturateOnIntegerOverflow=on  InputSameDT=on  OutDataTypeStr=Inherit: Same as first input
  Sum2 : Sum  Inputs=+-  SaturateOnIntegerOverflow=on  InputSameDT=on  OutDataTypeStr=Inherit: Same as first input
  Unit Delay1 : UnitDelay  SampleTime=Ts
  Unit Delay3 : UnitDelay  InitialCondition=Vc_Initial  SampleTime=Ts
  Unit Delay4 : UnitDelay  InitialCondition=Vc_Initial  SampleTime=Ts
  Vp : powerlib/Electrical Sources/Controlled Voltage Source  Initialize=off  Source_Type=AC  Amplitude=0  Phase=0  Frequency=0  Measurements=None
      settings: SourceProductName=Simscape Electrical
  Vp1 : powerlib/Electrical Sources/Controlled Voltage Source  Initialize=off  Source_Type=AC  Amplitude=0  Phase=0  Frequency=0  Measurements=None
      settings: SourceProductName=Simscape Electrical
  1 : PMIOPort  Side=Left
  2 : PMIOPort  Port=2  Side=Left
  Vc : Outport
  wires:
  N/1 -> Saturation1/1
  [Imod] -> Mux/1
  Unit Delay3/1 -> Sum2/2
  Unit Delay4/1 -> Unit Delay3/1, Gain2/1
  Gain2/1 -> Sum2/1
  Gain/1 -> Discrete-Time Integrator/1
  Discrete-Time Integrator/1 -> Unit Delay4/1
  Mux/1 -> Unit Delay1/1
  Product2/1 -> Demux/1
  Demux/1 -> [Vin]
  Demux/2 -> [Vbl]
  [Vin] -> Vp/1
  Current Measurement1/1 -> [Imod]
  Current Measurement2/1 -> [Icap]
  [Vbl] -> Vp1/1
  [Icap] -> Mux/2
  Unit Delay1/1 -> Product1/2
  Saturation1/1 -> Product1/1, Product2/1
  Product1/1 -> Sum1/1
  Sum2/1 -> Product2/2, Vc/1
  Sum1/1 -> Gain/1
  connections:
  1/RConn1 -- Vp/RConn1
  Vp/LConn1 -- Current Measurement1/LConn1
  Current Measurement1/RConn1 -- Dp/LConn1 -- Dp2/RConn1
  Current Measurement2/LConn1 -- Dp/RConn1
  Vp1/RConn1 -- Current Measurement2/RConn1
  Vp1/LConn1 -- 2/RConn1 -- Dp2/LConn1

== system clearing_faulted_segment_travelling_Wave/MMC Converter1/Half-Bridge MMC Ap2/HalfBridgeMMC_Agt_Discrete ==
  N : Inport  PortDimensions=2
  Current Measurement1 : powerlib/Measurements/Current Measurement  PhasorSimulation=off  OutputType=Complex  PSBequivalent=0
      settings: SourceProductName=Simscape Electrical
  Current Measurement2 : powerlib/Measurements/Current Measurement  PhasorSimulation=off  OutputType=Complex  PSBequivalent=0
      settings: SourceProductName=Simscape Electrical
  Demux : Demux  Outputs=2
  Discrete-Time Integrator : DiscreteIntegrator  IntegratorMethod=Integration: Trapezoidal  gainval=1  InitialCondition=Vc_Initial  SampleTime=Ts  UpperSaturationLimit=5000  LowerSaturationLimit=500  ICPrevOutput=DiscIntNeverNeededParam  ICPrevScaledInput=DiscIntNeverNeededParam
  Dp : powerlib/Power Electronics/Diode  Ron=Ron_Diode  Lon=0  Vf=Vf_Diode  IC=0  UseSnubber=off  Rs=Rs_Diode  Cs=Cs_Diode  Measurements=off
      settings: SourceProductName=Simscape Electrical
  Dp2 : powerlib/Power Electronics/Diode  Ron=Ron_Diode  Lon=0  Vf=Vf_Diode  IC=0  UseSnubber=off  Rs=Rs_Diode  Cs=Cs_Diode  Measurements=off
      settings: SourceProductName=Simscape Electrical
  Gain : Gain  Gain=1/(C*n)
  Gain2 : Gain  Gain=2
  Mux : Mux  Inputs=2
  Product1 : Product
  Product2 : Product
  Saturation1 : Saturate  UpperLimit=n  LowerLimit=0
  Sum1 : Sum  Inputs=1  SaturateOnIntegerOverflow=on  InputSameDT=on  OutDataTypeStr=Inherit: Same as first input
  Sum2 : Sum  Inputs=+-  SaturateOnIntegerOverflow=on  InputSameDT=on  OutDataTypeStr=Inherit: Same as first input
  Unit Delay1 : UnitDelay  SampleTime=Ts
  Unit Delay3 : UnitDelay  InitialCondition=Vc_Initial  SampleTime=Ts
  Unit Delay4 : UnitDelay  InitialCondition=Vc_Initial  SampleTime=Ts
  Vp : powerlib/Electrical Sources/Controlled Voltage Source  Initialize=off  Source_Type=AC  Amplitude=0  Phase=0  Frequency=0  Measurements=None
      settings: SourceProductName=Simscape Electrical
  Vp1 : powerlib/Electrical Sources/Controlled Voltage Source  Initialize=off  Source_Type=AC  Amplitude=0  Phase=0  Frequency=0  Measurements=None
      settings: SourceProductName=Simscape Electrical
  1 : PMIOPort  Side=Left
  2 : PMIOPort  Port=2  Side=Left
  Vc : Outport
  wires:
  Sum1/1 -> Gain/1
  Sum2/1 -> Vc/1, Product2/2
  Product1/1 -> Sum1/1
  Saturation1/1 -> Product2/1, Product1/1
  Unit Delay1/1 -> Product1/2
  [Icap] -> Mux/2
  [Vbl] -> Vp1/1
  Current Measurement2/1 -> [Icap]
  Current Measurement1/1 -> [Imod]
  [Vin] -> Vp/1
  Demux/2 -> [Vbl]
  Demux/1 -> [Vin]
  Product2/1 -> Demux/1
  Mux/1 -> Unit Delay1/1
  Discrete-Time Integrator/1 -> Unit Delay4/1
  Gain/1 -> Discrete-Time Integrator/1
  Gain2/1 -> Sum2/1
  Unit Delay4/1 -> Gain2/1, Unit Delay3/1
  Unit Delay3/1 -> Sum2/2
  [Imod] -> Mux/1
  N/1 -> Saturation1/1
  connections:
  Dp2/LConn1 -- 2/RConn1 -- Vp1/LConn1
  Vp1/RConn1 -- Current Measurement2/RConn1
  Current Measurement2/LConn1 -- Dp/RConn1
  Dp2/RConn1 -- Dp/LConn1 -- Current Measurement1/RConn1
  Vp/LConn1 -- Current Measurement1/LConn1
  1/RConn1 -- Vp/RConn1

== system clearing_faulted_segment_travelling_Wave/MMC Converter1/Half-Bridge MMC Ap3/HalfBridgeMMC_Agt_Discrete ==
  N : Inport  PortDimensions=2
  Current Measurement1 : powerlib/Measurements/Current Measurement  PhasorSimulation=off  OutputType=Complex  PSBequivalent=0
      settings: SourceProductName=Simscape Electrical
  Current Measurement2 : powerlib/Measurements/Current Measurement  PhasorSimulation=off  OutputType=Complex  PSBequivalent=0
      settings: SourceProductName=Simscape Electrical
  Demux : Demux  Outputs=2
  Discrete-Time Integrator : DiscreteIntegrator  IntegratorMethod=Integration: Trapezoidal  gainval=1  InitialCondition=Vc_Initial  SampleTime=Ts  UpperSaturationLimit=5000  LowerSaturationLimit=500  ICPrevOutput=DiscIntNeverNeededParam  ICPrevScaledInput=DiscIntNeverNeededParam
  Dp : powerlib/Power Electronics/Diode  Ron=Ron_Diode  Lon=0  Vf=Vf_Diode  IC=0  UseSnubber=off  Rs=Rs_Diode  Cs=Cs_Diode  Measurements=off
      settings: SourceProductName=Simscape Electrical
  Dp2 : powerlib/Power Electronics/Diode  Ron=Ron_Diode  Lon=0  Vf=Vf_Diode  IC=0  UseSnubber=off  Rs=Rs_Diode  Cs=Cs_Diode  Measurements=off
      settings: SourceProductName=Simscape Electrical
  Gain : Gain  Gain=1/(C*n)
  Gain2 : Gain  Gain=2
  Mux : Mux  Inputs=2
  Product1 : Product
  Product2 : Product
  Saturation1 : Saturate  UpperLimit=n  LowerLimit=0
  Sum1 : Sum  Inputs=1  SaturateOnIntegerOverflow=on  InputSameDT=on  OutDataTypeStr=Inherit: Same as first input
  Sum2 : Sum  Inputs=+-  SaturateOnIntegerOverflow=on  InputSameDT=on  OutDataTypeStr=Inherit: Same as first input
  Unit Delay1 : UnitDelay  SampleTime=Ts
  Unit Delay3 : UnitDelay  InitialCondition=Vc_Initial  SampleTime=Ts
  Unit Delay4 : UnitDelay  InitialCondition=Vc_Initial  SampleTime=Ts
  Vp : powerlib/Electrical Sources/Controlled Voltage Source  Initialize=off  Source_Type=AC  Amplitude=0  Phase=0  Frequency=0  Measurements=None
      settings: SourceProductName=Simscape Electrical
  Vp1 : powerlib/Electrical Sources/Controlled Voltage Source  Initialize=off  Source_Type=AC  Amplitude=0  Phase=0  Frequency=0  Measurements=None
      settings: SourceProductName=Simscape Electrical
  1 : PMIOPort  Side=Left
  2 : PMIOPort  Port=2  Side=Left
  Vc : Outport
  wires:
  Sum1/1 -> Gain/1
  Sum2/1 -> Vc/1, Product2/2
  Product1/1 -> Sum1/1
  Saturation1/1 -> Product2/1, Product1/1
  Unit Delay1/1 -> Product1/2
  [Icap] -> Mux/2
  [Vbl] -> Vp1/1
  Current Measurement2/1 -> [Icap]
  Current Measurement1/1 -> [Imod]
  [Vin] -> Vp/1
  Demux/2 -> [Vbl]
  Demux/1 -> [Vin]
  Product2/1 -> Demux/1
  Mux/1 -> Unit Delay1/1
  Discrete-Time Integrator/1 -> Unit Delay4/1
  Gain/1 -> Discrete-Time Integrator/1
  Gain2/1 -> Sum2/1
  Unit Delay4/1 -> Gain2/1, Unit Delay3/1
  Unit Delay3/1 -> Sum2/2
  [Imod] -> Mux/1
  N/1 -> Saturation1/1
  connections:
  Dp2/LConn1 -- 2/RConn1 -- Vp1/LConn1
  Vp1/RConn1 -- Current Measurement2/RConn1
  Current Measurement2/LConn1 -- Dp/RConn1
  Dp2/RConn1 -- Dp/LConn1 -- Current Measurement1/RConn1
  Vp/LConn1 -- Current Measurement1/LConn1
  1/RConn1 -- Vp/RConn1

== system clearing_faulted_segment_travelling_Wave/MMC Converter1/Half-Bridge MMC Ap4/HalfBridgeMMC_Agt_Discrete ==
  N : Inport  PortDimensions=2
  Current Measurement1 : powerlib/Measurements/Current Measurement  PhasorSimulation=off  OutputType=Complex  PSBequivalent=0
      settings: SourceProductName=Simscape Electrical
  Current Measurement2 : powerlib/Measurements/Current Measurement  PhasorSimulation=off  OutputType=Complex  PSBequivalent=0
      settings: SourceProductName=Simscape Electrical
  Demux : Demux  Outputs=2
  Discrete-Time Integrator : DiscreteIntegrator  IntegratorMethod=Integration: Trapezoidal  gainval=1  InitialCondition=Vc_Initial  SampleTime=Ts  UpperSaturationLimit=5000  LowerSaturationLimit=500  ICPrevOutput=DiscIntNeverNeededParam  ICPrevScaledInput=DiscIntNeverNeededParam
  Dp : powerlib/Power Electronics/Diode  Ron=Ron_Diode  Lon=0  Vf=Vf_Diode  IC=0  UseSnubber=off  Rs=Rs_Diode  Cs=Cs_Diode  Measurements=off
      settings: SourceProductName=Simscape Electrical
  Dp2 : powerlib/Power Electronics/Diode  Ron=Ron_Diode  Lon=0  Vf=Vf_Diode  IC=0  UseSnubber=off  Rs=Rs_Diode  Cs=Cs_Diode  Measurements=off
      settings: SourceProductName=Simscape Electrical
  Gain : Gain  Gain=1/(C*n)
  Gain2 : Gain  Gain=2
  Mux : Mux  Inputs=2
  Product1 : Product
  Product2 : Product
  Saturation1 : Saturate  UpperLimit=n  LowerLimit=0
  Sum1 : Sum  Inputs=1  SaturateOnIntegerOverflow=on  InputSameDT=on  OutDataTypeStr=Inherit: Same as first input
  Sum2 : Sum  Inputs=+-  SaturateOnIntegerOverflow=on  InputSameDT=on  OutDataTypeStr=Inherit: Same as first input
  Unit Delay1 : UnitDelay  SampleTime=Ts
  Unit Delay3 : UnitDelay  InitialCondition=Vc_Initial  SampleTime=Ts
  Unit Delay4 : UnitDelay  InitialCondition=Vc_Initial  SampleTime=Ts
  Vp : powerlib/Electrical Sources/Controlled Voltage Source  Initialize=off  Source_Type=AC  Amplitude=0  Phase=0  Frequency=0  Measurements=None
      settings: SourceProductName=Simscape Electrical
  Vp1 : powerlib/Electrical Sources/Controlled Voltage Source  Initialize=off  Source_Type=AC  Amplitude=0  Phase=0  Frequency=0  Measurements=None
      settings: SourceProductName=Simscape Electrical
  1 : PMIOPort  Side=Left
  2 : PMIOPort  Port=2  Side=Left
  Vc : Outport
  wires:
  N/1 -> Saturation1/1
  [Imod] -> Mux/1
  Unit Delay3/1 -> Sum2/2
  Unit Delay4/1 -> Unit Delay3/1, Gain2/1
  Gain2/1 -> Sum2/1
  Gain/1 -> Discrete-Time Integrator/1
  Discrete-Time Integrator/1 -> Unit Delay4/1
  Mux/1 -> Unit Delay1/1
  Product2/1 -> Demux/1
  Demux/1 -> [Vin]
  Demux/2 -> [Vbl]
  [Vin] -> Vp/1
  Current Measurement1/1 -> [Imod]
  Current Measurement2/1 -> [Icap]
  [Vbl] -> Vp1/1
  [Icap] -> Mux/2
  Unit Delay1/1 -> Product1/2
  Saturation1/1 -> Product1/1, Product2/1
  Product1/1 -> Sum1/1
  Sum2/1 -> Product2/2, Vc/1
  Sum1/1 -> Gain/1
  connections:
  1/RConn1 -- Vp/RConn1
  Vp/LConn1 -- Current Measurement1/LConn1
  Current Measurement1/RConn1 -- Dp/LConn1 -- Dp2/RConn1
  Current Measurement2/LConn1 -- Dp/RConn1
  Vp1/RConn1 -- Current Measurement2/RConn1
  Vp1/LConn1 -- 2/RConn1 -- Dp2/LConn1

== system clearing_faulted_segment_travelling_Wave/MMC Converter1/Half-Bridge MMC Ap5/HalfBridgeMMC_Agt_Discrete ==
  N : Inport  PortDimensions=2
  Current Measurement1 : powerlib/Measurements/Current Measurement  PhasorSimulation=off  OutputType=Complex  PSBequivalent=0
      settings: SourceProductName=Simscape Electrical
  Current Measurement2 : powerlib/Measurements/Current Measurement  PhasorSimulation=off  OutputType=Complex  PSBequivalent=0
      settings: SourceProductName=Simscape Electrical
  Demux : Demux  Outputs=2
  Discrete-Time Integrator : DiscreteIntegrator  IntegratorMethod=Integration: Trapezoidal  gainval=1  InitialCondition=Vc_Initial  SampleTime=Ts  UpperSaturationLimit=5000  LowerSaturationLimit=500  ICPrevOutput=DiscIntNeverNeededParam  ICPrevScaledInput=DiscIntNeverNeededParam
  Dp : powerlib/Power Electronics/Diode  Ron=Ron_Diode  Lon=0  Vf=Vf_Diode  IC=0  UseSnubber=off  Rs=Rs_Diode  Cs=Cs_Diode  Measurements=off
      settings: SourceProductName=Simscape Electrical
  Dp2 : powerlib/Power Electronics/Diode  Ron=Ron_Diode  Lon=0  Vf=Vf_Diode  IC=0  UseSnubber=off  Rs=Rs_Diode  Cs=Cs_Diode  Measurements=off
      settings: SourceProductName=Simscape Electrical
  Gain : Gain  Gain=1/(C*n)
  Gain2 : Gain  Gain=2
  Mux : Mux  Inputs=2
  Product1 : Product
  Product2 : Product
  Saturation1 : Saturate  UpperLimit=n  LowerLimit=0
  Sum1 : Sum  Inputs=1  SaturateOnIntegerOverflow=on  InputSameDT=on  OutDataTypeStr=Inherit: Same as first input
  Sum2 : Sum  Inputs=+-  SaturateOnIntegerOverflow=on  InputSameDT=on  OutDataTypeStr=Inherit: Same as first input
  Unit Delay1 : UnitDelay  SampleTime=Ts
  Unit Delay3 : UnitDelay  InitialCondition=Vc_Initial  SampleTime=Ts
  Unit Delay4 : UnitDelay  InitialCondition=Vc_Initial  SampleTime=Ts
  Vp : powerlib/Electrical Sources/Controlled Voltage Source  Initialize=off  Source_Type=AC  Amplitude=0  Phase=0  Frequency=0  Measurements=None
      settings: SourceProductName=Simscape Electrical
  Vp1 : powerlib/Electrical Sources/Controlled Voltage Source  Initialize=off  Source_Type=AC  Amplitude=0  Phase=0  Frequency=0  Measurements=None
      settings: SourceProductName=Simscape Electrical
  1 : PMIOPort  Side=Left
  2 : PMIOPort  Port=2  Side=Left
  Vc : Outport
  wires:
  Sum1/1 -> Gain/1
  Sum2/1 -> Vc/1, Product2/2
  Product1/1 -> Sum1/1
  Saturation1/1 -> Product2/1, Product1/1
  Unit Delay1/1 -> Product1/2
  [Icap] -> Mux/2
  [Vbl] -> Vp1/1
  Current Measurement2/1 -> [Icap]
  Current Measurement1/1 -> [Imod]
  [Vin] -> Vp/1
  Demux/2 -> [Vbl]
  Demux/1 -> [Vin]
  Product2/1 -> Demux/1
  Mux/1 -> Unit Delay1/1
  Discrete-Time Integrator/1 -> Unit Delay4/1
  Gain/1 -> Discrete-Time Integrator/1
  Gain2/1 -> Sum2/1
  Unit Delay4/1 -> Gain2/1, Unit Delay3/1
  Unit Delay3/1 -> Sum2/2
  [Imod] -> Mux/1
  N/1 -> Saturation1/1
  connections:
  Dp2/LConn1 -- 2/RConn1 -- Vp1/LConn1
  Vp1/RConn1 -- Current Measurement2/RConn1
  Current Measurement2/LConn1 -- Dp/RConn1
  Dp2/RConn1 -- Dp/LConn1 -- Current Measurement1/RConn1
  Vp/LConn1 -- Current Measurement1/LConn1
  1/RConn1 -- Vp/RConn1

== system clearing_faulted_segment_travelling_Wave/MMC Converter2/Half-Bridge MMC Ap/HalfBridgeMMC_Agt_Discrete ==
  N : Inport  PortDimensions=2
  Current Measurement1 : powerlib/Measurements/Current Measurement  PhasorSimulation=off  OutputType=Complex  PSBequivalent=0
      settings: SourceProductName=Simscape Electrical
  Current Measurement2 : powerlib/Measurements/Current Measurement  PhasorSimulation=off  OutputType=Complex  PSBequivalent=0
      settings: SourceProductName=Simscape Electrical
  Demux : Demux  Outputs=2
  Discrete-Time Integrator : DiscreteIntegrator  IntegratorMethod=Integration: Trapezoidal  gainval=1  InitialCondition=Vc_Initial  SampleTime=Ts  UpperSaturationLimit=5000  LowerSaturationLimit=500  ICPrevOutput=DiscIntNeverNeededParam  ICPrevScaledInput=DiscIntNeverNeededParam
  Dp : powerlib/Power Electronics/Diode  Ron=Ron_Diode  Lon=0  Vf=Vf_Diode  IC=0  UseSnubber=off  Rs=Rs_Diode  Cs=Cs_Diode  Measurements=off
      settings: SourceProductName=Simscape Electrical
  Dp2 : powerlib/Power Electronics/Diode  Ron=Ron_Diode  Lon=0  Vf=Vf_Diode  IC=0  UseSnubber=off  Rs=Rs_Diode  Cs=Cs_Diode  Measurements=off
      settings: SourceProductName=Simscape Electrical
  Gain : Gain  Gain=1/(C*n)
  Gain2 : Gain  Gain=2
  Mux : Mux  Inputs=2
  Product1 : Product
  Product2 : Product
  Saturation1 : Saturate  UpperLimit=n  LowerLimit=0
  Sum1 : Sum  Inputs=1  SaturateOnIntegerOverflow=on  InputSameDT=on  OutDataTypeStr=Inherit: Same as first input
  Sum2 : Sum  Inputs=+-  SaturateOnIntegerOverflow=on  InputSameDT=on  OutDataTypeStr=Inherit: Same as first input
  Unit Delay1 : UnitDelay  SampleTime=Ts
  Unit Delay3 : UnitDelay  InitialCondition=Vc_Initial  SampleTime=Ts
  Unit Delay4 : UnitDelay  InitialCondition=Vc_Initial  SampleTime=Ts
  Vp : powerlib/Electrical Sources/Controlled Voltage Source  Initialize=off  Source_Type=AC  Amplitude=0  Phase=0  Frequency=0  Measurements=None
      settings: SourceProductName=Simscape Electrical
  Vp1 : powerlib/Electrical Sources/Controlled Voltage Source  Initialize=off  Source_Type=AC  Amplitude=0  Phase=0  Frequency=0  Measurements=None
      settings: SourceProductName=Simscape Electrical
  1 : PMIOPort  Side=Left
  2 : PMIOPort  Port=2  Side=Left
  Vc : Outport
  wires:
  N/1 -> Saturation1/1
  [Imod] -> Mux/1
  Unit Delay3/1 -> Sum2/2
  Unit Delay4/1 -> Unit Delay3/1, Gain2/1
  Gain2/1 -> Sum2/1
  Gain/1 -> Discrete-Time Integrator/1
  Discrete-Time Integrator/1 -> Unit Delay4/1
  Mux/1 -> Unit Delay1/1
  Product2/1 -> Demux/1
  Demux/1 -> [Vin]
  Demux/2 -> [Vbl]
  [Vin] -> Vp/1
  Current Measurement1/1 -> [Imod]
  Current Measurement2/1 -> [Icap]
  [Vbl] -> Vp1/1
  [Icap] -> Mux/2
  Unit Delay1/1 -> Product1/2
  Saturation1/1 -> Product1/1, Product2/1
  Product1/1 -> Sum1/1
  Sum2/1 -> Product2/2, Vc/1
  Sum1/1 -> Gain/1
  connections:
  1/RConn1 -- Vp/RConn1
  Vp/LConn1 -- Current Measurement1/LConn1
  Current Measurement1/RConn1 -- Dp/LConn1 -- Dp2/RConn1
  Current Measurement2/LConn1 -- Dp/RConn1
  Vp1/RConn1 -- Current Measurement2/RConn1
  Vp1/LConn1 -- 2/RConn1 -- Dp2/LConn1

== system clearing_faulted_segment_travelling_Wave/MMC Converter2/Half-Bridge MMC Ap1/HalfBridgeMMC_Agt_Discrete ==
  N : Inport  PortDimensions=2
  Current Measurement1 : powerlib/Measurements/Current Measurement  PhasorSimulation=off  OutputType=Complex  PSBequivalent=0
      settings: SourceProductName=Simscape Electrical
  Current Measurement2 : powerlib/Measurements/Current Measurement  PhasorSimulation=off  OutputType=Complex  PSBequivalent=0
      settings: SourceProductName=Simscape Electrical
  Demux : Demux  Outputs=2
  Discrete-Time Integrator : DiscreteIntegrator  IntegratorMethod=Integration: Trapezoidal  gainval=1  InitialCondition=Vc_Initial  SampleTime=Ts  UpperSaturationLimit=5000  LowerSaturationLimit=500  ICPrevOutput=DiscIntNeverNeededParam  ICPrevScaledInput=DiscIntNeverNeededParam
  Dp : powerlib/Power Electronics/Diode  Ron=Ron_Diode  Lon=0  Vf=Vf_Diode  IC=0  UseSnubber=off  Rs=Rs_Diode  Cs=Cs_Diode  Measurements=off
      settings: SourceProductName=Simscape Electrical
  Dp2 : powerlib/Power Electronics/Diode  Ron=Ron_Diode  Lon=0  Vf=Vf_Diode  IC=0  UseSnubber=off  Rs=Rs_Diode  Cs=Cs_Diode  Measurements=off
      settings: SourceProductName=Simscape Electrical
  Gain : Gain  Gain=1/(C*n)
  Gain2 : Gain  Gain=2
  Mux : Mux  Inputs=2
  Product1 : Product
  Product2 : Product
  Saturation1 : Saturate  UpperLimit=n  LowerLimit=0
  Sum1 : Sum  Inputs=1  SaturateOnIntegerOverflow=on  InputSameDT=on  OutDataTypeStr=Inherit: Same as first input
  Sum2 : Sum  Inputs=+-  SaturateOnIntegerOverflow=on  InputSameDT=on  OutDataTypeStr=Inherit: Same as first input
  Unit Delay1 : UnitDelay  SampleTime=Ts
  Unit Delay3 : UnitDelay  InitialCondition=Vc_Initial  SampleTime=Ts
  Unit Delay4 : UnitDelay  InitialCondition=Vc_Initial  SampleTime=Ts
  Vp : powerlib/Electrical Sources/Controlled Voltage Source  Initialize=off  Source_Type=AC  Amplitude=0  Phase=0  Frequency=0  Measurements=None
      settings: SourceProductName=Simscape Electrical
  Vp1 : powerlib/Electrical Sources/Controlled Voltage Source  Initialize=off  Source_Type=AC  Amplitude=0  Phase=0  Frequency=0  Measurements=None
      settings: SourceProductName=Simscape Electrical
  1 : PMIOPort  Side=Left
  2 : PMIOPort  Port=2  Side=Left
  Vc : Outport
  wires:
  N/1 -> Saturation1/1
  [Imod] -> Mux/1
  Unit Delay3/1 -> Sum2/2
  Unit Delay4/1 -> Unit Delay3/1, Gain2/1
  Gain2/1 -> Sum2/1
  Gain/1 -> Discrete-Time Integrator/1
  Discrete-Time Integrator/1 -> Unit Delay4/1
  Mux/1 -> Unit Delay1/1
  Product2/1 -> Demux/1
  Demux/1 -> [Vin]
  Demux/2 -> [Vbl]
  [Vin] -> Vp/1
  Current Measurement1/1 -> [Imod]
  Current Measurement2/1 -> [Icap]
  [Vbl] -> Vp1/1
  [Icap] -> Mux/2
  Unit Delay1/1 -> Product1/2
  Saturation1/1 -> Product1/1, Product2/1
  Product1/1 -> Sum1/1
  Sum2/1 -> Product2/2, Vc/1
  Sum1/1 -> Gain/1
  connections:
  1/RConn1 -- Vp/RConn1
  Vp/LConn1 -- Current Measurement1/LConn1
  Current Measurement1/RConn1 -- Dp/LConn1 -- Dp2/RConn1
  Current Measurement2/LConn1 -- Dp/RConn1
  Vp1/RConn1 -- Current Measurement2/RConn1
  Vp1/LConn1 -- 2/RConn1 -- Dp2/LConn1
